simulink model "linear_model"  (Simulink 7.6)
settings: Solver=FixedStepDiscrete  StartTime=0.0  StopTime=2  FixedStep=0.001  RelTol=1e-3
undefined symbols (not defined in the file): C, D, F, G, Gamma, H, K, Phi, Ts, x0
settings Model: Creator=Fodi  LastModifiedBy=Fodi

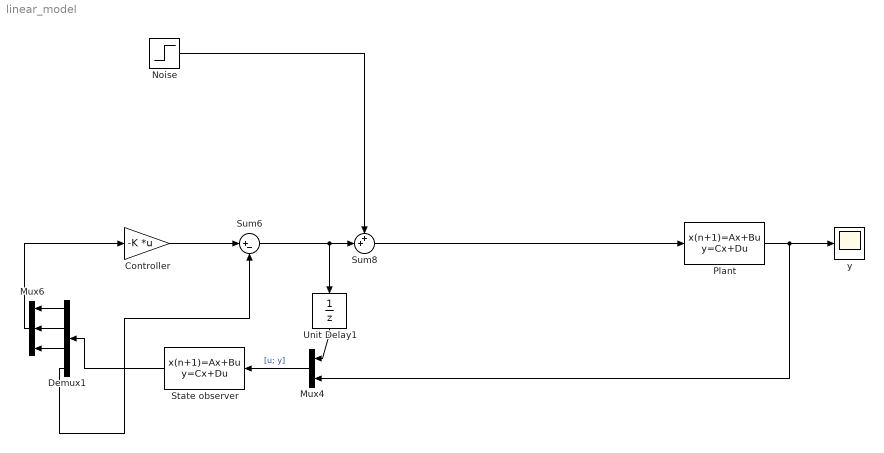
== system linear_model ==
  Controller : Gain  Gain=-K  Multiplication=Matrix(K*u)
  Demux1 : Demux
  Mux4 : Mux  Inputs=2
  Mux6 : Mux  Inputs=3
  Noise : Step  Time=5  After=0  SampleTime=Ts
  Plant : DiscreteStateSpace  A=Phi  B=Gamma  C=C  D=D  X0=x0  SampleTime=Ts
  State observer : DiscreteStateSpace  A=F  B=[H G]  C=eye(size(F))  D=zeros(size(F,1),size([H G],2))  SampleTime=Ts
  Sum6 : Sum  Inputs=|+-
  Sum8 : Sum  Inputs=++|
  Unit Delay1 : UnitDelay  SampleTime=-1
  y : Scope
      settings: TimeRange=10  YMin=-0.002  YMax=0.012  SaveName=y2
  wires:
  Sum6/1 -> Sum8/2, Unit Delay1/1
  Plant/1 -> y/1, Mux4/2
  Mux4/1 -> State observer/1  "[u; y]"
  Noise/1 -> Sum8/1
  Mux6/1 -> Controller/1
  Demux1/1 -> Mux6/1
  Demux1/2 -> Mux6/2
  Demux1/3 -> Mux6/3
  State observer/1 -> Demux1/1
  Unit Delay1/1 -> Mux4/1
  Controller/1 -> Sum6/1
  Demux1/4 -> Sum6/2
  Sum8/1 -> Plant/1
